simulink model "gm_parallel_8_min_cost_function"  (R2022a)
settings: Solver=FixedStepDiscrete  StartTime=0.0  StopTime=10.0  RelTol=1e-3
undefined symbols (not defined in the file or in its folder): f_c
libraries: hdlmdlgenlib x40
(part 1 of 2)
settings Model: Creator=Andre Merx  LastModifiedBy=Andre Merx
settings SolverCC: AlgebraicLoopSolver=TrustRegion
settings DataIOCC: LimitDataPoints=on  SaveOutput=off  SaveTime=off
settings OptimizationCC: BlockReduction=off  ConditionallyExecuteInputs=off  DefaultParameterBehavior=Inlined  LifeSpan=inf
settings DebuggingCC: AlgebraicLoopMsg=error  InheritedTsInSrcMsg=none  SingleTaskRateTransMsg=error  UnconnectedInputMsg=warning  UnconnectedOutputMsg=warning  UnconnectedLineMsg=warning  AllowSymbolicDim=off  StrictBusMsg=ErrorOnBusTreatedAsVector  SFUnexpectedBacktrackingDiag=warning  SFNoUnconditionalDefaultTransitionDiag=warning  SFExecutionAtInitializationDiag=none  SFMachineParentedDataDiag=warning  ArithmeticOperatorsInVariantConditions=warning
settings HardwareCC: ProdBitPerPointer=32  ProdBitPerSizeT=32  ProdBitPerPtrDiffT=32  ProdLargestAtomicFloat=None  ProdIntDivRoundTo=Undefined  ProdEndianess=Unspecified  ProdWordSize=32  ProdHWDeviceType=ASIC/FPGA->ASIC/FPGA  ProdEqTarget=off
settings SFSimCC: SimUseLocalCustomCode=off  CustomCodeUndefinedFunction=UseInterfaceOnly
settings RTWCC: RTWUseLocalCustomCode=off
settings CodeAppCC: StateflowObjectComments=on
settings GRTTargetCC: TargetLangStandard=C89/C90 (ANSI)
settings ConfigComp: CovScope=ReferencedModels  CovMetricSettings=dw  CovSaveCumulativeToWorkspaceVar=on  CovSaveSingleToWorkspaceVar=on  CovExternalEMLEnable=off  CovSFcnEnable=off

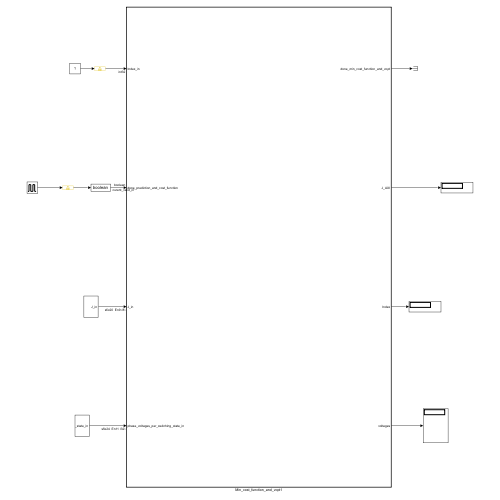
[thumbnail: Simulink's stored preview of the top-level diagram]
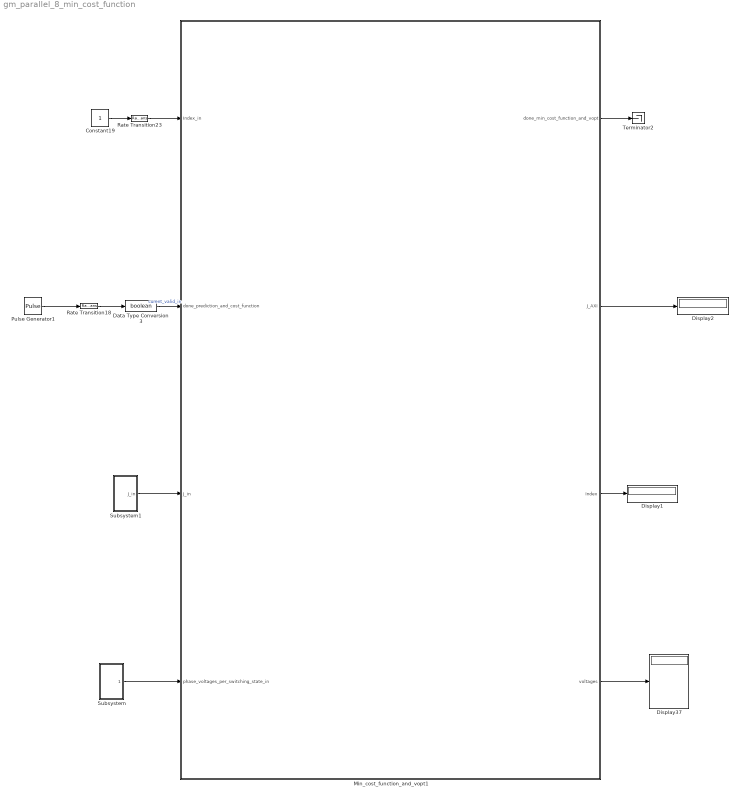
== system gm_parallel_8_min_cost_function ==
  Constant19 : Constant  OutDataTypeStr=int32  SampleTime=-1
  Data Type Conversion3 : DataTypeConversion  OutDataTypeStr=boolean  SaturateOnIntegerOverflow=off  RndMeth=Floor
  Display1 : Display
  Display2 : Display
  Display37 : Display
  Min_cost_function_and_vopt1 : Subsystem  TreatAsAtomicUnit=on
  Pulse Generator1 : DiscretePulseGenerator  PulseType=Time based  Period=1/f_c
  Rate Transition18 : RateTransition  OutPortSampleTime=Rt
  Rate Transition23 : RateTransition  OutPortSampleTime=Rt
  Subsystem : Subsystem
  Subsystem1 : Subsystem
  Terminator2 : Terminator
  wires:
  Min_cost_function_and_vopt1/1(done_min_cost_function_and_vopt) -> Terminator2/1
  Min_cost_function_and_vopt1/2(J_AXI) -> Display2/1
  Min_cost_function_and_vopt1/3(Index) -> Display1/1
  Min_cost_function_and_vopt1/4(voltages) -> Display37/1
  Rate Transition18/1 -> Data Type Conversion3/1
  Pulse Generator1/1 -> Rate Transition18/1
  Data Type Conversion3/1 -> Min_cost_function_and_vopt1/2(done_prediction_and_cost_function)  "curent_valid_in"
  Rate Transition23/1 -> Min_cost_function_and_vopt1/1(Index_in)
  Constant19/1 -> Rate Transition23/1
  Subsystem1/1(J_in) -> Min_cost_function_and_vopt1/3(J_in)
  Subsystem/1(phase_voltages_per_switching_state_in) -> Min_cost_function_and_vopt1/4(phase_voltages_per_switching_state_in)

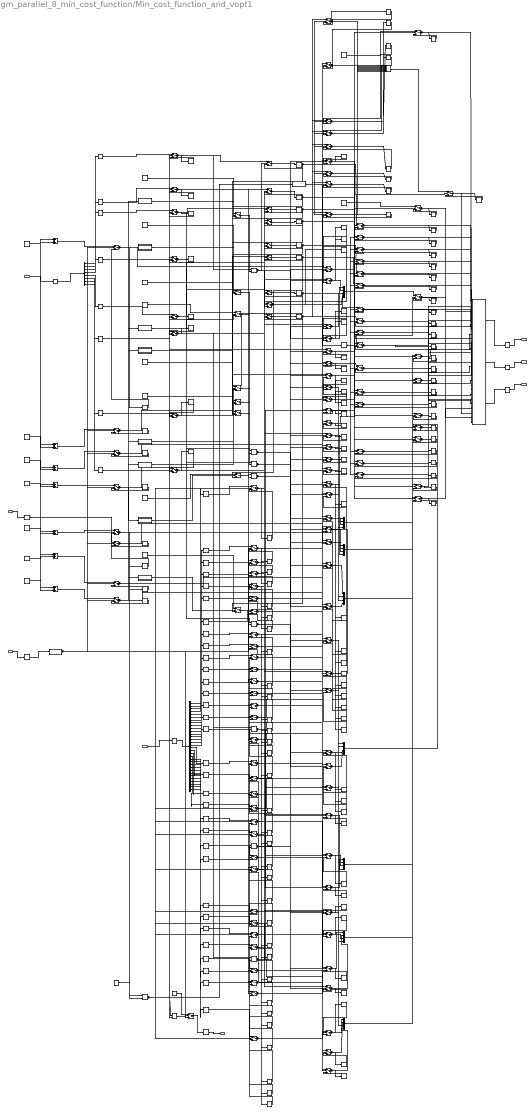
== system gm_parallel_8_min_cost_function/Min_cost_function_and_vopt1 ==
  Index_in : Inport  OutDataTypeStr=int32  PortDimensions=1  SampleTime=1e-08
  done_prediction_and_cost_function : Inport  Port=2  OutDataTypeStr=boolean  PortDimensions=1  SampleTime=1e-08
  J_in : Inport  Port=3  OutDataTypeStr=fixdt(1, 20, 9)  PortDimensions=[8]  SampleTime=1e-08
  phase_voltages_per_switching_state_in : Inport  Port=4  OutDataTypeStr=fixdt(1, 24, 11)  PortDimensions=[32]  SampleTime=1e-08
  Add{,1..6} (7 alike) : Sum  AccumDataTypeStr=fixdt(1, 33, 0)  OutDataTypeStr=fixdt(1, 33, 0)  SampleTime=1e-08
  Compare To Constant : Subsystem  mask(Compare To Constant){relop=<=, const=double(1), OutDataTypeStr=boolean, ZeroCross=on}
      mask prompts: relop "Simulink:masks:Operator_MP"; const "Simulink:masks:ConstantValue_MP"; OutDataTypeStr "Simulink:masks:OutputDataType_MP"; ZeroCross "Simulink:masks:EnableZerocrossingDetection_MP"
      mask help: Simulink:masks:CompareToConstant_MD
      mask init:
      | OutDataTypeStr = 'boolean';
      | ZeroCross = 'on';
      | blkName = 'parallel_8_min_cost_function/Min_cost_function_and_vopt1/Compare\nTo Constant';
      | const = double(1);
      | const_str = '1';
      | const_val = double(1);
      | relop = '<=';
      | setValue = 'boolean';
      | str = '<= 1';
      mask TypeOptions relop: == | ~= | < | <= | >= | >
      mask TypeOptions OutDataTypeStr: Simulink:masks:uint8 | Simulink:masks:boolean
      mask Callback ZeroCross: sl('zeroCrossEnable', gcbh);
      mask Display: disp(str)
  Compare To Constant1 : Subsystem  mask(Compare To Constant){relop=<=, const=double(9), OutDataTypeStr=boolean, ZeroCross=on}
      mask prompts: relop "Simulink:masks:Operator_MP"; const "Simulink:masks:ConstantValue_MP"; OutDataTypeStr "Simulink:masks:OutputDataType_MP"; ZeroCross "Simulink:masks:EnableZerocrossingDetection_MP"
      mask help: Simulink:masks:CompareToConstant_MD
      mask init:
      | OutDataTypeStr = 'boolean';
      | ZeroCross = 'on';
      | blkName = 'parallel_8_min_cost_function/Min_cost_function_and_vopt1/Compare\nTo Constant1';
      | const = double(9);
      | const_str = '9';
      | const_val = double(9);
      | relop = '<=';
      | setValue = 'boolean';
      | str = '<= 9';
      mask TypeOptions relop: == | ~= | < | <= | >= | >
      mask TypeOptions OutDataTypeStr: Simulink:masks:uint8 | Simulink:masks:boolean
      mask Callback ZeroCross: sl('zeroCrossEnable', gcbh);
      mask Display: disp(str)
  Compare To Constant2 : Subsystem  mask(Compare To Constant){relop=<=, const=double(17), OutDataTypeStr=boolean, ZeroCross=on}
      mask prompts: relop "Simulink:masks:Operator_MP"; const "Simulink:masks:ConstantValue_MP"; OutDataTypeStr "Simulink:masks:OutputDataType_MP"; ZeroCross "Simulink:masks:EnableZerocrossingDetection_MP"
      mask help: Simulink:masks:CompareToConstant_MD
      mask init:
      | OutDataTypeStr = 'boolean';
      | ZeroCross = 'on';
      | blkName = 'parallel_8_min_cost_function/Min_cost_function_and_vopt1/Compare\nTo Constant2';
      | const = double(17);
      | const_str = '17';
      | const_val = double(17);
      | relop = '<=';
      | setValue = 'boolean';
      | str = '<= 17';
      mask TypeOptions relop: == | ~= | < | <= | >= | >
      mask TypeOptions OutDataTypeStr: Simulink:masks:uint8 | Simulink:masks:boolean
      mask Callback ZeroCross: sl('zeroCrossEnable', gcbh);
      mask Display: disp(str)
  Compare To Constant3 : Subsystem  mask(Compare To Constant){relop=<=, const=double(25), OutDataTypeStr=boolean, ZeroCross=on}
      mask prompts: relop "Simulink:masks:Operator_MP"; const "Simulink:masks:ConstantValue_MP"; OutDataTypeStr "Simulink:masks:OutputDataType_MP"; ZeroCross "Simulink:masks:EnableZerocrossingDetection_MP"
      mask help: Simulink:masks:CompareToConstant_MD
      mask init:
      | OutDataTypeStr = 'boolean';
      | ZeroCross = 'on';
      | blkName = 'parallel_8_min_cost_function/Min_cost_function_and_vopt1/Compare\nTo Constant3';
      | const = double(25);
      | const_str = '25';
      | const_val = double(25);
      | relop = '<=';
      | setValue = 'boolean';
      | str = '<= 25';
      mask TypeOptions relop: == | ~= | < | <= | >= | >
      mask TypeOptions OutDataTypeStr: Simulink:masks:uint8 | Simulink:masks:boolean
      mask Callback ZeroCross: sl('zeroCrossEnable', gcbh);
      mask Display: disp(str)
  Compare To Constant4 : Subsystem  mask(Compare To Constant){relop=<=, const=double(33), OutDataTypeStr=boolean, ZeroCross=on}
      mask prompts: relop "Simulink:masks:Operator_MP"; const "Simulink:masks:ConstantValue_MP"; OutDataTypeStr "Simulink:masks:OutputDataType_MP"; ZeroCross "Simulink:masks:EnableZerocrossingDetection_MP"
      mask help: Simulink:masks:CompareToConstant_MD
      mask init:
      | OutDataTypeStr = 'boolean';
      | ZeroCross = 'on';
      | blkName = 'parallel_8_min_cost_function/Min_cost_function_and_vopt1/Compare\nTo Constant4';
      | const = double(33);
      | const_str = '33';
      | const_val = double(33);
      | relop = '<=';
      | setValue = 'boolean';
      | str = '<= 33';
      mask TypeOptions relop: == | ~= | < | <= | >= | >
      mask TypeOptions OutDataTypeStr: Simulink:masks:uint8 | Simulink:masks:boolean
      mask Callback ZeroCross: sl('zeroCrossEnable', gcbh);
      mask Display: disp(str)
  Compare To Constant5 : Subsystem  mask(Compare To Constant){relop=<=, const=double(41), OutDataTypeStr=boolean, ZeroCross=on}
      mask prompts: relop "Simulink:masks:Operator_MP"; const "Simulink:masks:ConstantValue_MP"; OutDataTypeStr "Simulink:masks:OutputDataType_MP"; ZeroCross "Simulink:masks:EnableZerocrossingDetection_MP"
      mask help: Simulink:masks:CompareToConstant_MD
      mask init:
      | OutDataTypeStr = 'boolean';
      | ZeroCross = 'on';
      | blkName = 'parallel_8_min_cost_function/Min_cost_function_and_vopt1/Compare\nTo Constant5';
      | const = double(41);
      | const_str = '41';
      | const_val = double(41);
      | relop = '<=';
      | setValue = 'boolean';
      | str = '<= 41';
      mask TypeOptions relop: == | ~= | < | <= | >= | >
      mask TypeOptions OutDataTypeStr: Simulink:masks:uint8 | Simulink:masks:boolean
      mask Callback ZeroCross: sl('zeroCrossEnable', gcbh);
      mask Display: disp(str)
  Compare To Constant6 : Subsystem  mask(Compare To Constant){relop=<=, const=double(49), OutDataTypeStr=boolean, ZeroCross=on}
      mask prompts: relop "Simulink:masks:Operator_MP"; const "Simulink:masks:ConstantValue_MP"; OutDataTypeStr "Simulink:masks:OutputDataType_MP"; ZeroCross "Simulink:masks:EnableZerocrossingDetection_MP"
      mask help: Simulink:masks:CompareToConstant_MD
      mask init:
      | OutDataTypeStr = 'boolean';
      | ZeroCross = 'on';
      | blkName = 'parallel_8_min_cost_function/Min_cost_function_and_vopt1/Compare\nTo Constant6';
      | const = double(49);
      | const_str = '49';
      | const_val = double(49);
      | relop = '<=';
      | setValue = 'boolean';
      | str = '<= 49';
      mask TypeOptions relop: == | ~= | < | <= | >= | >
      mask TypeOptions OutDataTypeStr: Simulink:masks:uint8 | Simulink:masks:boolean
      mask Callback ZeroCross: sl('zeroCrossEnable', gcbh);
      mask Display: disp(str)
  Compare To Constant7 : Subsystem  mask(Compare To Constant){relop=<=, const=double(57), OutDataTypeStr=boolean, ZeroCross=on}
      mask prompts: relop "Simulink:masks:Operator_MP"; const "Simulink:masks:ConstantValue_MP"; OutDataTypeStr "Simulink:masks:OutputDataType_MP"; ZeroCross "Simulink:masks:EnableZerocrossingDetection_MP"
      mask help: Simulink:masks:CompareToConstant_MD
      mask init:
      | OutDataTypeStr = 'boolean';
      | ZeroCross = 'on';
      | blkName = 'parallel_8_min_cost_function/Min_cost_function_and_vopt1/Compare\nTo Constant7';
      | const = double(57);
      | const_str = '57';
      | const_val = double(57);
      | relop = '<=';
      | setValue = 'boolean';
      | str = '<= 57';
      mask TypeOptions relop: == | ~= | < | <= | >= | >
      mask TypeOptions OutDataTypeStr: Simulink:masks:uint8 | Simulink:masks:boolean
      mask Callback ZeroCross: sl('zeroCrossEnable', gcbh);
      mask Display: disp(str)
  Constant{,3..9} (8 alike) : Constant  Value=1000  OutDataTypeStr=fixdt(1, 20, 9)  SampleTime=1e-08
  Constant1 : Constant  Value=8  OutDataTypeStr=int32  SampleTime=1e-08
  Constant10 : Constant  Value=0  OutDataTypeStr=fixdt(1, 20, 9)  SampleTime=1e-08
  Constant11 : Constant  Value="repmat(0,[4  1])"  OutDataTypeStr=fixdt(1, 24, 11)  SampleTime=1e-08
  Constant18 : Constant  Value=8  OutDataTypeStr=int32  SampleTime=1e-08
  Constant19 : Constant  Value=16  OutDataTypeStr=int32  SampleTime=1e-08
  Constant2 : Constant  Value=0  OutDataTypeStr=boolean  SampleTime=1e-08
  Constant20 : Constant  Value=24  OutDataTypeStr=int32  SampleTime=1e-08
  Constant21 : Constant  Value=32  OutDataTypeStr=int32  SampleTime=1e-08
  Constant22 : Constant  Value=40  OutDataTypeStr=int32  SampleTime=1e-08
  Constant23 : Constant  Value=48  OutDataTypeStr=int32  SampleTime=1e-08
  Constant24 : Constant  Value=56  OutDataTypeStr=int32  SampleTime=1e-08
  Delay{,1..9,11..73,81..90,95..96,104..113,118..119,127..136,141..142,150..159,164..165,173..182,371..378} (139 alike) : Delay  DelayLength=double(1)  InitialCondition=0  SampleTime=1e-08
  Delay74 : Delay  DelayLength=double(2)  InitialCondition=0  SampleTime=1e-08
  Delay7_out1_0_wire : hdlmdlgenlib/Buffer
      settings: SourceProductBaseCode=SL
  Delay7_out1_1_wire : hdlmdlgenlib/Buffer
      settings: SourceProductBaseCode=SL
  Delay7_out1_2_wire : hdlmdlgenlib/Buffer
      settings: SourceProductBaseCode=SL
  Delay7_out1_3_wire : hdlmdlgenlib/Buffer
      settings: SourceProductBaseCode=SL
  Delay7_out1_4_wire : hdlmdlgenlib/Buffer
      settings: SourceProductBaseCode=SL
  Delay7_out1_5_wire : hdlmdlgenlib/Buffer
      settings: SourceProductBaseCode=SL
  Delay7_out1_6_wire : hdlmdlgenlib/Buffer
      settings: SourceProductBaseCode=SL
  Delay7_out1_7_wire : hdlmdlgenlib/Buffer
      settings: SourceProductBaseCode=SL
  Delay8_out1_0_wire : hdlmdlgenlib/Buffer
      settings: SourceProductBaseCode=SL
  Delay8_out1_10_wire : hdlmdlgenlib/Buffer
      settings: SourceProductBaseCode=SL
  Delay8_out1_11_wire : hdlmdlgenlib/Buffer
      settings: SourceProductBaseCode=SL
  Delay8_out1_12_wire : hdlmdlgenlib/Buffer
      settings: SourceProductBaseCode=SL
  Delay8_out1_13_wire : hdlmdlgenlib/Buffer
      settings: SourceProductBaseCode=SL
  Delay8_out1_14_wire : hdlmdlgenlib/Buffer
      settings: SourceProductBaseCode=SL
  Delay8_out1_15_wire : hdlmdlgenlib/Buffer
      settings: SourceProductBaseCode=SL
  Delay8_out1_16_wire : hdlmdlgenlib/Buffer
      settings: SourceProductBaseCode=SL
  Delay8_out1_17_wire : hdlmdlgenlib/Buffer
      settings: SourceProductBaseCode=SL
  Delay8_out1_18_wire : hdlmdlgenlib/Buffer
      settings: SourceProductBaseCode=SL
  Delay8_out1_19_wire : hdlmdlgenlib/Buffer
      settings: SourceProductBaseCode=SL
  Delay8_out1_1_wire : hdlmdlgenlib/Buffer
      settings: SourceProductBaseCode=SL
  Delay8_out1_20_wire : hdlmdlgenlib/Buffer
      settings: SourceProductBaseCode=SL
  Delay8_out1_21_wire : hdlmdlgenlib/Buffer
      settings: SourceProductBaseCode=SL
  Delay8_out1_22_wire : hdlmdlgenlib/Buffer
      settings: SourceProductBaseCode=SL
  Delay8_out1_23_wire : hdlmdlgenlib/Buffer
      settings: SourceProductBaseCode=SL
  Delay8_out1_24_wire : hdlmdlgenlib/Buffer
      settings: SourceProductBaseCode=SL
  Delay8_out1_25_wire : hdlmdlgenlib/Buffer
      settings: SourceProductBaseCode=SL
  Delay8_out1_26_wire : hdlmdlgenlib/Buffer
      settings: SourceProductBaseCode=SL
  Delay8_out1_27_wire : hdlmdlgenlib/Buffer
      settings: SourceProductBaseCode=SL
  Delay8_out1_28_wire : hdlmdlgenlib/Buffer
      settings: SourceProductBaseCode=SL
  Delay8_out1_29_wire : hdlmdlgenlib/Buffer
      settings: SourceProductBaseCode=SL
  Delay8_out1_2_wire : hdlmdlgenlib/Buffer
      settings: SourceProductBaseCode=SL
  Delay8_out1_30_wire : hdlmdlgenlib/Buffer
      settings: SourceProductBaseCode=SL
  Delay8_out1_31_wire : hdlmdlgenlib/Buffer
      settings: SourceProductBaseCode=SL
  Delay8_out1_3_wire : hdlmdlgenlib/Buffer
      settings: SourceProductBaseCode=SL
  Delay8_out1_4_wire : hdlmdlgenlib/Buffer
      settings: SourceProductBaseCode=SL
  Delay8_out1_5_wire : hdlmdlgenlib/Buffer
      settings: SourceProductBaseCode=SL
  Delay8_out1_6_wire : hdlmdlgenlib/Buffer
      settings: SourceProductBaseCode=SL
  Delay8_out1_7_wire : hdlmdlgenlib/Buffer
      settings: SourceProductBaseCode=SL
  Delay8_out1_8_wire : hdlmdlgenlib/Buffer
      settings: SourceProductBaseCode=SL
  Delay8_out1_9_wire : hdlmdlgenlib/Buffer
      settings: SourceProductBaseCode=SL
  Detect Rise Positive : Subsystem  mask(Detect Rise Positive){vinit=double(0), InputProcessing=Elements as channels (sample based), OutDataTypeStr=boolean}
      mask prompts: vinit "Simulink:masks:InitialCondition_MP"; InputProcessing "Simulink:masks:InputProcessing_MP"; OutDataTypeStr "Simulink:masks:OutputDataType_MP"
      mask help: Simulink:masks:DetectRisePositive_MD
      mask init:
      | InputProcessing = 'Elements as channels (sample based)';
      | OutDataTypeStr = 'boolean';
      | vinit = double(0);
      mask TypeOptions InputProcessing: Simulink:masks:ColumnsAsChannelsFrameBased | Simulink:masks:ElementsAsChannelsSampleBased
      mask TypeOptions OutDataTypeStr: Simulink:masks:uint8 | Simulink:masks:boolean
      mask Display: fprintf('U > 0\n&  NOT\nU/z > 0')
  Detect Rise Positive1 : Subsystem  mask(Detect Rise Positive){vinit=double(0), InputProcessing=Elements as channels (sample based), OutDataTypeStr=boolean}
      mask prompts: vinit "Simulink:masks:InitialCondition_MP"; InputProcessing "Simulink:masks:InputProcessing_MP"; OutDataTypeStr "Simulink:masks:OutputDataType_MP"
      mask help: Simulink:masks:DetectRisePositive_MD
      mask init:
      | InputProcessing = 'Elements as channels (sample based)';
      | OutDataTypeStr = 'boolean';
      | vinit = double(0);
      mask TypeOptions InputProcessing: Simulink:masks:ColumnsAsChannelsFrameBased | Simulink:masks:ElementsAsChannelsSampleBased
      mask TypeOptions OutDataTypeStr: Simulink:masks:uint8 | Simulink:masks:boolean
      mask Display: fprintf('U > 0\n&  NOT\nU/z > 0')
  Logical Operator : Logic  AllPortsSameDT=off  OutDataTypeStr=boolean  SampleTime=1e-08
  MATLAB Function : Subsystem
  MinMax : MinMax  Inputs=8  ZeroCross=off
  Relational Operator{,2..8} (8 alike) : RelationalOperator  Operator=<  OutDataTypeStr=boolean  SampleTime=1e-08  InputSameDT=off
  Relational Operator1 : RelationalOperator  Operator===  OutDataTypeStr=boolean  SampleTime=1e-08  InputSameDT=off
  Switch{,1,8..9,20..21,27..28,34..35,41..42,48..49,55..56} (16 alike) : Switch  Criteria=u2 > Threshold  Threshold=double(0)  OutDataTypeStr=fixdt(1, 20, 9)  SampleTime=1e-08  SaturateOnIntegerOverflow=off  InputSameDT=off
  Switch{2,10,15,22,29,36,43,50} (8 alike) : Switch  Criteria=u2 > Threshold  Threshold=double(0)  OutDataTypeStr=int32  SampleTime=1e-08  SaturateOnIntegerOverflow=off  InputSameDT=off
  Switch{3..6,11..14,16..19,23..26,30..33,37..40,44..47,51..54} (32 alike) : Switch  Criteria=u2 > Threshold  Threshold=double(0)  OutDataTypeStr=fixdt(1, 24, 11)  SampleTime=1e-08  SaturateOnIntegerOverflow=off  InputSameDT=off
  Switch7 : Switch  Criteria=u2 > Threshold  Threshold=double(0)  OutDataTypeStr=boolean  SampleTime=1e-08  SaturateOnIntegerOverflow=off  InputSameDT=off
  Switch_on{1,53,56,59,62,65,68,71,74} (9 alike) : Switch  Threshold=double(1)  OutDataTypeStr=int32  RndMeth=Simplest  SampleTime=1e-08  SaturateOnIntegerOverflow=off  InputSameDT=off
  Switch_on{4,10,14,20,26,32,38,44,50..51,54,57,60,63,66,69,72,75,98..105} (26 alike) : Switch  Threshold=double(1)  OutDataTypeStr=fixdt(1, 20, 9)  RndMeth=Simplest  SampleTime=1e-08  SaturateOnIntegerOverflow=off  InputSameDT=off
  Switch_on{2..3,5..6,8..9,11..13,15..16,18..19,21..22,24..25,27..28,30..31,33..34,36..37,39..40,42..43,45..46,48..49,52,55,58,61,64,67,70,73} (41 alike) : Switch  Threshold=double(1)  OutDataTypeStr=fixdt(1, 24, 11)  RndMeth=Simplest  SampleTime=1e-08  SaturateOnIntegerOverflow=off  InputSameDT=off
  Switch_on{7,17,23,29,35,41,47} (7 alike) : Switch  Threshold=double(1)  OutDataTypeStr=fixdt(1, 33, 0)  RndMeth=Simplest  SampleTime=1e-08  SaturateOnIntegerOverflow=off  InputSameDT=off
  mux{,1..7} (8 alike) : Mux
  t : Demux  Outputs=8
  t1 : Demux  Outputs=32
  done_min_cost_function_and_vopt : Outport  SampleTime=1e-08
  J_AXI : Outport  Port=2  SampleTime=1e-08
  Index : Outport  Port=3  SampleTime=1e-08
  voltages : Outport  Port=4  SampleTime=1e-08
  wires:
  Index_in/1 -> Delay9/1
  done_prediction_and_cost_function/1 -> Delay6/1
  J_in/1 -> Delay7/1
  phase_voltages_per_switching_state_in/1 -> Delay8/1
  Add/1 -> Switch_on7/1
  Add1/1 -> Switch_on17/1
  Add2/1 -> Switch_on23/1
  Add3/1 -> Switch_on29/1
  Add4/1 -> Switch_on35/1
  Add5/1 -> Switch_on41/1
  Add6/1 -> Switch_on47/1
  Compare To Constant/1(y) -> Switch/2
  Compare To Constant1/1(y) -> Switch8/2
  Compare To Constant2/1(y) -> Switch20/2
  Compare To Constant3/1(y) -> Switch27/2
  Compare To Constant4/1(y) -> Switch34/2
  Compare To Constant5/1(y) -> Switch41/2
  Compare To Constant6/1(y) -> Switch48/2
  Compare To Constant7/1(y) -> Switch55/2
  Constant/1 -> Switch/1
  Constant1/1 -> Relational Operator1/1
  Constant10/1 -> Switch_on50/1
  Constant11/1 -> Switch_on13/1
  Constant18/1 -> Add/2
  Constant19/1 -> Add1/2
  Constant2/1 -> Switch7/1
  Constant20/1 -> Add2/2
  Constant21/1 -> Add3/2
  Constant22/1 -> Add4/2
  Constant23/1 -> Add5/2
  Constant24/1 -> Add6/2
  Constant3/1 -> Switch8/1
  Constant4/1 -> Switch20/1
  Constant5/1 -> Switch27/1
  Constant6/1 -> Switch34/1
  Constant7/1 -> Switch41/1
  Constant8/1 -> Switch48/1
  Constant9/1 -> Switch55/1
  Delay/1 -> Switch_on98/1, Switch_on75/1, Switch1/3, Switch/3
  Delay1/1 -> Switch2/3
  Delay104/1 -> Switch_on26/3
  Delay105/1 -> Switch_on29/3
  Delay106/1 -> Switch_on30/3
  Delay107/1 -> Switch30/3
  Delay108/1 -> Switch_on31/3
  Delay109/1 -> Switch_on27/3
  Delay11/1 -> done_min_cost_function_and_vopt/1
  Delay110/1 -> Switch_on28/3
  Delay111/1 -> Switch31/3
  Delay112/1 -> Switch32/3
  Delay113/1 -> Switch33/3
  Delay118/1 -> Switch_on60/1, Switch_on105/1, Switch42/3, Switch41/3
  Delay119/1 -> Switch36/3
  Delay12/1 -> voltages/1
  Delay127/1 -> Switch_on32/3
  Delay128/1 -> Switch_on35/3
  Delay129/1 -> Switch_on36/3
  Delay13/1 -> Index/1
  Delay130/1 -> Switch37/3
  Delay131/1 -> Switch_on37/3
  Delay132/1 -> Switch_on33/3
  Delay133/1 -> Switch_on34/3
  Delay134/1 -> Switch38/3
  Delay135/1 -> Switch39/3
  Delay136/1 -> Switch40/3
  Delay14/1 -> J_AXI/1
  Delay141/1 -> Switch_on57/1, Switch_on102/1, Switch49/3, Switch48/3
  Delay142/1 -> Switch43/3
  Delay15/1 -> Switch_on13/3
  Delay150/1 -> Switch_on38/3
  Delay151/1 -> Switch_on41/3
  Delay152/1 -> Switch_on42/3
  Delay153/1 -> Switch44/3
  Delay154/1 -> Switch_on43/3
  Delay155/1 -> Switch_on39/3
  Delay156/1 -> Switch_on40/3
  Delay157/1 -> Switch45/3
  Delay158/1 -> Switch46/3
  Delay159/1 -> Switch47/3
  Delay16/1 -> Switch_on50/3
  Delay164/1 -> Switch_on54/1, Switch_on103/1, Switch56/3, Switch55/3
  Delay165/1 -> Switch50/3
  Delay17/1 -> Switch_on4/3
  Delay173/1 -> Switch_on44/3
  Delay174/1 -> Switch_on47/3
  Delay175/1 -> Switch_on48/3
  Delay176/1 -> Switch51/3
  Delay177/1 -> Switch_on49/3
  Delay178/1 -> Switch_on45/3
  Delay179/1 -> Switch_on46/3
  Delay18/1 -> Switch_on1/3
  Delay180/1 -> Switch52/3
  Delay181/1 -> Switch53/3
  Delay182/1 -> Switch54/3
  Delay19/1 -> Switch_on2/3
  Delay2/1 -> Switch3/3
  Delay20/1 -> Switch_on3/3
  Delay21/1 -> Switch_on5/3
  Delay22/1 -> Switch_on6/3
  Delay23/1 -> Switch_on51/3
  Delay24/1 -> Switch_on52/3
  Delay25/1 -> Switch_on99/1, Switch_on72/1, Switch9/3, Switch8/3
  Delay26/1 -> Switch10/3
  Delay27/1 -> Switch_on53/3
  Delay28/1 -> Switch_on54/3
  Delay29/1 -> Switch_on55/3
  Delay3/1 -> Switch4/3
  Delay30/1 -> Switch_on56/3
  Delay31/1 -> Switch_on57/3
  Delay32/1 -> Switch_on58/3
  Delay33/1 -> Switch_on59/3
  Delay34/1 -> Switch_on10/3
  Delay35/1 -> Switch_on7/3
  Delay36/1 -> Switch_on8/3
  Delay37/1 -> Switch11/3
  Delay371/1 -> Switch_on98/3
  Delay372/1 -> Switch_on99/3
  Delay373/1 -> Switch_on100/3
  Delay374/1 -> Switch_on101/3
  Delay375/1 -> Switch_on104/3
  Delay376/1 -> Switch_on105/3
  Delay377/1 -> Switch_on102/3
  Delay378/1 -> Switch_on103/3
  Delay38/1 -> Switch_on9/3
  Delay39/1 -> Switch_on11/3
  Delay4/1 -> Switch5/3
  Delay40/1 -> Switch_on12/3
  Delay41/1 -> Switch12/3
  Delay42/1 -> Switch13/3
  Delay43/1 -> Switch14/3
  Delay44/1 -> Switch_on60/3
  Delay45/1 -> Switch_on61/3
  Delay46/1 -> Switch_on62/3
  Delay47/1 -> Switch_on63/3
  Delay48/1 -> Switch_on64/3
  Delay49/1 -> Switch_on69/1, Switch_on100/1, Switch21/3, Switch20/3
  Delay5/1 -> Switch6/3
  Delay50/1 -> Switch15/3
  Delay51/1 -> Switch_on65/3
  Delay52/1 -> Switch_on66/3
  Delay53/1 -> Switch_on67/3
  Delay54/1 -> Switch_on68/3
  Delay55/1 -> Switch_on69/3
  Delay56/1 -> Switch_on70/3
  Delay57/1 -> Switch_on71/3
  Delay58/1 -> Switch_on14/3
  Delay59/1 -> Switch_on17/3
  Delay6/1 -> Detect Rise Positive/1(U)
  Delay60/1 -> Switch_on18/3
  Delay61/1 -> Switch16/3
  Delay62/1 -> Switch_on19/3
  Delay63/1 -> Switch_on15/3
  Delay64/1 -> Switch_on16/3
  Delay65/1 -> Switch17/3
  Delay66/1 -> Switch18/3
  Delay67/1 -> Switch19/3
  Delay68/1 -> Switch_on72/3
  Delay69/1 -> Switch_on73/3
  Delay7/1 -> t/1
  Delay70/1 -> Switch_on74/3
  Delay71/1 -> Switch_on75/3
  Delay72/1 -> Switch_on66/1, Switch_on101/1, Switch28/3, Switch27/3
  Delay73/1 -> Switch22/3
  Delay74/1 -> Switch_on75/2, Switch_on74/2, Switch_on73/2, Switch_on72/2, Switch_on71/2, Switch_on70/2, Switch_on69/2, Switch_on68/2, Switch_on67/2, Switch_on66/2, Switch_on65/2, Switch_on64/2, Switch_on63/2, Switch_on62/2, Switch_on61/2, Switch_on60/2, Switch_on59/2, Switch_on58/2, Switch_on57/2, Switch_on56/2, Switch_on55/2, Switch_on54/2, Switch_on53/2, Switch_on52/2, Switch_on51/2, Switch_on50/2, Switch_on13/2
  Delay8/1 -> t1/1
  Delay81/1 -> Switch_on20/3
  Delay82/1 -> Switch_on23/3
  Delay83/1 -> Switch_on24/3
  Delay84/1 -> Switch23/3
  Delay85/1 -> Switch_on25/3
  Delay86/1 -> Switch_on21/3
  Delay87/1 -> Switch_on22/3
  Delay88/1 -> Switch24/3
  Delay89/1 -> Switch25/3
  Delay9/1 -> Switch_on1/1, Add6/1, Add5/1, Add4/1, Add3/1, Add2/1, Add1/1, Add/1
  Delay90/1 -> Switch26/3
  Delay95/1 -> Switch_on63/1, Switch_on104/1, Switch35/3, Switch34/3
  Delay96/1 -> Switch29/3
  Delay7_out1_0_wire/1 -> Switch_on4/1
  Delay7_out1_1_wire/1 -> Switch_on10/1
  Delay7_out1_2_wire/1 -> Switch_on14/1
  Delay7_out1_3_wire/1 -> Switch_on20/1
  Delay7_out1_4_wire/1 -> Switch_on26/1
  Delay7_out1_5_wire/1 -> Switch_on32/1
  Delay7_out1_6_wire/1 -> Switch_on38/1
  Delay7_out1_7_wire/1 -> Switch_on44/1
  Delay8_out1_0_wire/1 -> Switch_on2/1
  Delay8_out1_1_wire/1 -> Switch_on3/1
  Delay8_out1_2_wire/1 -> Switch_on5/1
  Delay8_out1_3_wire/1 -> Switch_on6/1
  Delay8_out1_4_wire/1 -> Switch_on8/1
  Delay8_out1_5_wire/1 -> Switch_on9/1
  Delay8_out1_6_wire/1 -> Switch_on11/1
  Delay8_out1_7_wire/1 -> Switch_on12/1
  Delay8_out1_8_wire/1 -> Switch_on18/1
  Delay8_out1_9_wire/1 -> Switch_on19/1
  Delay8_out1_10_wire/1 -> Switch_on15/1
  Delay8_out1_11_wire/1 -> Switch_on16/1
  Delay8_out1_12_wire/1 -> Switch_on24/1
  Delay8_out1_13_wire/1 -> Switch_on25/1
  Delay8_out1_14_wire/1 -> Switch_on21/1
  Delay8_out1_15_wire/1 -> Switch_on22/1
  Delay8_out1_16_wire/1 -> Switch_on30/1
  Delay8_out1_17_wire/1 -> Switch_on31/1
  Delay8_out1_18_wire/1 -> Switch_on27/1
  Delay8_out1_19_wire/1 -> Switch_on28/1
  Delay8_out1_20_wire/1 -> Switch_on36/1
  Delay8_out1_21_wire/1 -> Switch_on37/1
  Delay8_out1_22_wire/1 -> Switch_on33/1
  Delay8_out1_23_wire/1 -> Switch_on34/1
  Delay8_out1_24_wire/1 -> Switch_on42/1
  Delay8_out1_25_wire/1 -> Switch_on43/1
  Delay8_out1_26_wire/1 -> Switch_on39/1
  Delay8_out1_27_wire/1 -> Switch_on40/1
  Delay8_out1_28_wire/1 -> Switch_on48/1
  Delay8_out1_29_wire/1 -> Switch_on49/1
  Delay8_out1_30_wire/1 -> Switch_on45/1
  Delay8_out1_31_wire/1 -> Switch_on46/1
  Detect Rise Positive/1(Y) -> Switch_on9/2, Switch_on8/2, Switch_on7/2, Switch_on6/2, Switch_on5/2, Switch_on49/2, Switch_on48/2, Switch_on47/2, Switch_on46/2, Switch_on45/2, Switch_on44/2, Switch_on43/2, Switch_on42/2, Switch_on41/2, Switch_on40/2, Switch_on4/2, Switch_on39/2, Switch_on38/2, Switch_on37/2, Switch_on36/2, Switch_on35/2, Switch_on34/2, Switch_on33/2, Switch_on32/2, Switch_on31/2, Switch_on30/2, Switch_on3/2, Switch_on29/2, Switch_on28/2, Switch_on27/2, Switch_on26/2, Switch_on25/2, Switch_on24/2, Switch_on23/2, Switch_on22/2, Switch_on21/2, Switch_on20/2, Switch_on2/2, Switch_on19/2, Switch_on18/2, Switch_on17/2, Switch_on16/2, Switch_on15/2, Switch_on14/2, Switch_on12/2, Switch_on11/2, Switch_on10/2, Switch_on1/2, Switch7/3, Logical Operator/2
  Detect Rise Positive1/1(Y) -> Switch_on99/2, Switch_on98/2, Switch_on105/2, Switch_on104/2, Switch_on103/2, Switch_on102/2, Switch_on101/2, Switch_on100/2, Delay74/1
  Logical Operator/1 -> Switch7/2
  MATLAB Function/1(J) -> Delay14/1
  MATLAB Function/2(Index) -> Delay13/1
  MATLAB Function/3(voltages) -> Delay12/1
  MinMax/1 -> Switch_on51/1
  mux/1 -> Switch_on73/1
  mux1/1 -> Switch_on70/1
  mux2/1 -> Switch_on67/1
  mux3/1 -> Switch_on64/1
  mux4/1 -> Switch_on61/1
  mux5/1 -> Switch_on58/1
  mux6/1 -> Switch_on55/1
  mux7/1 -> Switch_on52/1
  Relational Operator/1 -> Switch6/2, Switch5/2, Switch4/2, Switch3/2, Switch2/2, Switch1/2
  Relational Operator1/1 -> Logical Operator/1, Detect Rise Positive1/1(U)
  Relational Operator2/1 -> Switch9/2, Switch14/2, Switch13/2, Switch12/2, Switch11/2, Switch10/2
  Relational Operator3/1 -> Switch21/2, Switch19/2, Switch18/2, Switch17/2, Switch16/2, Switch15/2
  Relational Operator4/1 -> Switch28/2, Switch26/2, Switch25/2, Switch24/2, Switch23/2, Switch22/2
  Relational Operator5/1 -> Switch35/2, Switch33/2, Switch32/2, Switch31/2, Switch30/2, Switch29/2
  Relational Operator6/1 -> Switch42/2, Switch40/2, Switch39/2, Switch38/2, Switch37/2, Switch36/2
  Relational Operator7/1 -> Switch49/2, Switch47/2, Switch46/2, Switch45/2, Switch44/2, Switch43/2
  Relational Operator8/1 -> Switch56/2, Switch54/2, Switch53/2, Switch52/2, Switch51/2, Switch50/2
  Switch/1 -> Relational Operator/2
  Switch1/1 -> Delay/1
  Switch10/1 -> Switch_on71/1, Delay26/1
  Switch11/1 -> mux1/1, Delay37/1
  Switch12/1 -> mux1/2, Delay41/1
  Switch13/1 -> mux1/3, Delay42/1
  Switch14/1 -> mux1/4, Delay43/1
  Switch15/1 -> Switch_on68/1, Delay50/1
  Switch16/1 -> mux2/1, Delay61/1
  Switch17/1 -> mux2/2, Delay65/1
  Switch18/1 -> mux2/3, Delay66/1
  Switch19/1 -> mux2/4, Delay67/1
  Switch2/1 -> Switch_on74/1, Delay1/1
  Switch20/1 -> Relational Operator3/2
  Switch21/1 -> Delay49/1
  Switch22/1 -> Switch_on65/1, Delay73/1
  Switch23/1 -> mux3/1, Delay84/1
  Switch24/1 -> mux3/2, Delay88/1
  Switch25/1 -> mux3/3, Delay89/1
  Switch26/1 -> mux3/4, Delay90/1
  Switch27/1 -> Relational Operator4/2
  Switch28/1 -> Delay72/1
  Switch29/1 -> Switch_on62/1, Delay96/1
  Switch3/1 -> mux/1, Delay2/1
  Switch30/1 -> mux4/1, Delay107/1
  Switch31/1 -> mux4/2, Delay111/1
  Switch32/1 -> mux4/3, Delay112/1
  Switch33/1 -> mux4/4, Delay113/1
  Switch34/1 -> Relational Operator5/2
  Switch35/1 -> Delay95/1
  Switch36/1 -> Switch_on59/1, Delay119/1
  Switch37/1 -> mux5/1, Delay130/1
  Switch38/1 -> mux5/2, Delay134/1
  Switch39/1 -> mux5/3, Delay135/1
  Switch4/1 -> mux/2, Delay3/1
  Switch40/1 -> mux5/4, Delay136/1
  Switch41/1 -> Relational Operator6/2
  Switch42/1 -> Delay118/1
  Switch43/1 -> Switch_on56/1, Delay142/1
  Switch44/1 -> mux6/1, Delay153/1
  Switch45/1 -> mux6/2, Delay157/1
  Switch46/1 -> mux6/3, Delay158/1
  Switch47/1 -> mux6/4, Delay159/1
  Switch48/1 -> Relational Operator7/2
  Switch49/1 -> Delay141/1
  Switch5/1 -> mux/3, Delay4/1
  Switch50/1 -> Switch_on53/1, Delay165/1
  Switch51/1 -> mux7/1, Delay176/1
  Switch52/1 -> mux7/2, Delay180/1
  Switch53/1 -> mux7/3, Delay181/1
  Switch54/1 -> mux7/4, Delay182/1
  Switch55/1 -> Relational Operator8/2
  Switch56/1 -> Delay164/1
  Switch6/1 -> mux/4, Delay5/1
  Switch7/1 -> Delay11/1
  Switch8/1 -> Relational Operator2/2
  Switch9/1 -> Delay25/1
  Switch_on1/1 -> Switch2/1, Relational Operator1/2, Delay18/1, Compare To Constant/1(u)
  Switch_on10/1 -> Switch9/1, Relational Operator2/1, Delay34/1
  Switch_on100/1 -> Delay373/1, MinMax/3
  Switch_on101/1 -> Delay374/1, MinMax/4
  Switch_on102/1 -> Delay377/1, MinMax/7
  Switch_on103/1 -> Delay378/1, MinMax/8
  Switch_on104/1 -> Delay375/1, MinMax/5
  Switch_on105/1 -> Delay376/1, MinMax/6
  Switch_on11/1 -> Switch13/1, Delay39/1
  Switch_on12/1 -> Switch14/1, Delay40/1
  Switch_on13/1 -> Delay15/1, MATLAB Function/27(voltages_default)
  Switch_on14/1 -> Switch21/1, Relational Operator3/1, Delay58/1
  Switch_on15/1 -> Switch18/1, Delay63/1
  Switch_on16/1 -> Switch19/1, Delay64/1
  Switch_on17/1 -> Switch15/1, Delay59/1, Compare To Constant2/1(u)
  Switch_on18/1 -> Switch16/1, Delay60/1
  Switch_on19/1 -> Switch17/1, Delay62/1
  Switch_on2/1 -> Switch3/1, Delay19/1
  Switch_on20/1 -> Switch28/1, Relational Operator4/1, Delay81/1
  Switch_on21/1 -> Switch25/1, Delay86/1
  Switch_on22/1 -> Switch26/1, Delay87/1
  Switch_on23/1 -> Switch22/1, Delay82/1, Compare To Constant3/1(u)
  Switch_on24/1 -> Switch23/1, Delay83/1
  Switch_on25/1 -> Switch24/1, Delay85/1
  Switch_on26/1 -> Switch35/1, Relational Operator5/1, Delay104/1
  Switch_on27/1 -> Switch32/1, Delay109/1
  Switch_on28/1 -> Switch33/1, Delay110/1
  Switch_on29/1 -> Switch29/1, Delay105/1, Compare To Constant4/1(u)
  Switch_on3/1 -> Switch4/1, Delay20/1
  Switch_on30/1 -> Switch30/1, Delay106/1
  Switch_on31/1 -> Switch31/1, Delay108/1
  Switch_on32/1 -> Switch42/1, Relational Operator6/1, Delay127/1
  Switch_on33/1 -> Switch39/1, Delay132/1
  Switch_on34/1 -> Switch40/1, Delay133/1
  Switch_on35/1 -> Switch36/1, Delay128/1, Compare To Constant5/1(u)
  Switch_on36/1 -> Switch37/1, Delay129/1
  Switch_on37/1 -> Switch38/1, Delay131/1
  Switch_on38/1 -> Switch49/1, Relational Operator7/1, Delay150/1
  Switch_on39/1 -> Switch46/1, Delay155/1
  Switch_on4/1 -> Switch1/1, Relational Operator/1, Delay17/1
  Switch_on40/1 -> Switch47/1, Delay156/1
  Switch_on41/1 -> Switch43/1, Delay151/1, Compare To Constant6/1(u)
  Switch_on42/1 -> Switch44/1, Delay152/1
  Switch_on43/1 -> Switch45/1, Delay154/1
  Switch_on44/1 -> Switch56/1, Relational Operator8/1, Delay173/1
  Switch_on45/1 -> Switch53/1, Delay178/1
  Switch_on46/1 -> Switch54/1, Delay179/1
  Switch_on47/1 -> Switch50/1, Delay174/1, Compare To Constant7/1(u)
  Switch_on48/1 -> Switch51/1, Delay175/1
  Switch_on49/1 -> Switch52/1, Delay177/1
  Switch_on5/1 -> Switch5/1, Delay21/1
  Switch_on50/1 -> Delay16/1, MATLAB Function/26(J_default)
  Switch_on51/1 -> Delay23/1, MATLAB Function/25(min)
  Switch_on52/1 -> Delay24/1, MATLAB Function/24(voltages_8)
  Switch_on53/1 -> Delay27/1, MATLAB Function/23(Index_8)
  Switch_on54/1 -> Delay28/1, MATLAB Function/22(J_8)
  Switch_on55/1 -> Delay29/1, MATLAB Function/21(voltages_7)
  Switch_on56/1 -> Delay30/1, MATLAB Function/20(Index_7)
  Switch_on57/1 -> Delay31/1, MATLAB Function/19(J_7)
  Switch_on58/1 -> Delay32/1, MATLAB Function/18(voltages_6)
  Switch_on59/1 -> Delay33/1, MATLAB Function/17(Index_6)
  Switch_on6/1 -> Switch6/1, Delay22/1
  Switch_on60/1 -> Delay44/1, MATLAB Function/16(J_6)
  Switch_on61/1 -> Delay45/1, MATLAB Function/15(voltages_5)
  Switch_on62/1 -> Delay46/1, MATLAB Function/14(Index_5)
  Switch_on63/1 -> Delay47/1, MATLAB Function/13(J_5)
  Switch_on64/1 -> Delay48/1, MATLAB Function/12(voltages_4)
  Switch_on65/1 -> Delay51/1, MATLAB Function/11(Index_4)
  Switch_on66/1 -> Delay52/1, MATLAB Function/10(J_4)
  Switch_on67/1 -> Delay53/1, MATLAB Function/9(voltages_3)
  Switch_on68/1 -> Delay54/1, MATLAB Function/8(Index_3)
  Switch_on69/1 -> Delay55/1, MATLAB Function/7(J_3)
  Switch_on7/1 -> Switch10/1, Delay35/1, Compare To Constant1/1(u)
  Switch_on70/1 -> Delay56/1, MATLAB Function/6(voltages_2)
  Switch_on71/1 -> Delay57/1, MATLAB Function/5(Index_2)
  Switch_on72/1 -> Delay68/1, MATLAB Function/4(J_2)
  Switch_on73/1 -> Delay69/1, MATLAB Function/3(voltages_1)
  Switch_on74/1 -> Delay70/1, MATLAB Function/2(Index_1)
  Switch_on75/1 -> Delay71/1, MATLAB Function/1(J_1)
  Switch_on8/1 -> Switch11/1, Delay36/1
  Switch_on9/1 -> Switch12/1, Delay38/1
  Switch_on98/1 -> Delay371/1, MinMax/1
  Switch_on99/1 -> Delay372/1, MinMax/2
  t/1 -> Delay7_out1_0_wire/1
  t/2 -> Delay7_out1_1_wire/1
  t/3 -> Delay7_out1_2_wire/1
  t/4 -> Delay7_out1_3_wire/1
  t/5 -> Delay7_out1_4_wire/1
  t/6 -> Delay7_out1_5_wire/1
  t/7 -> Delay7_out1_6_wire/1
  t/8 -> Delay7_out1_7_wire/1
  t1/1 -> Delay8_out1_0_wire/1
  t1/2 -> Delay8_out1_1_wire/1
  t1/3 -> Delay8_out1_2_wire/1
  t1/4 -> Delay8_out1_3_wire/1
  t1/5 -> Delay8_out1_4_wire/1
  t1/6 -> Delay8_out1_5_wire/1
  t1/7 -> Delay8_out1_6_wire/1
  t1/8 -> Delay8_out1_7_wire/1
  t1/9 -> Delay8_out1_8_wire/1
  t1/10 -> Delay8_out1_9_wire/1
  t1/11 -> Delay8_out1_10_wire/1
  t1/12 -> Delay8_out1_11_wire/1
  t1/13 -> Delay8_out1_12_wire/1
  t1/14 -> Delay8_out1_13_wire/1
  t1/15 -> Delay8_out1_14_wire/1
  t1/16 -> Delay8_out1_15_wire/1
  t1/17 -> Delay8_out1_16_wire/1
  t1/18 -> Delay8_out1_17_wire/1
  t1/19 -> Delay8_out1_18_wire/1
  t1/20 -> Delay8_out1_19_wire/1
  t1/21 -> Delay8_out1_20_wire/1
  t1/22 -> Delay8_out1_21_wire/1
  t1/23 -> Delay8_out1_22_wire/1
  t1/24 -> Delay8_out1_23_wire/1
  t1/25 -> Delay8_out1_24_wire/1
  t1/26 -> Delay8_out1_25_wire/1
  t1/27 -> Delay8_out1_26_wire/1
  t1/28 -> Delay8_out1_27_wire/1
  t1/29 -> Delay8_out1_28_wire/1
  t1/30 -> Delay8_out1_29_wire/1
  t1/31 -> Delay8_out1_30_wire/1
  t1/32 -> Delay8_out1_31_wire/1

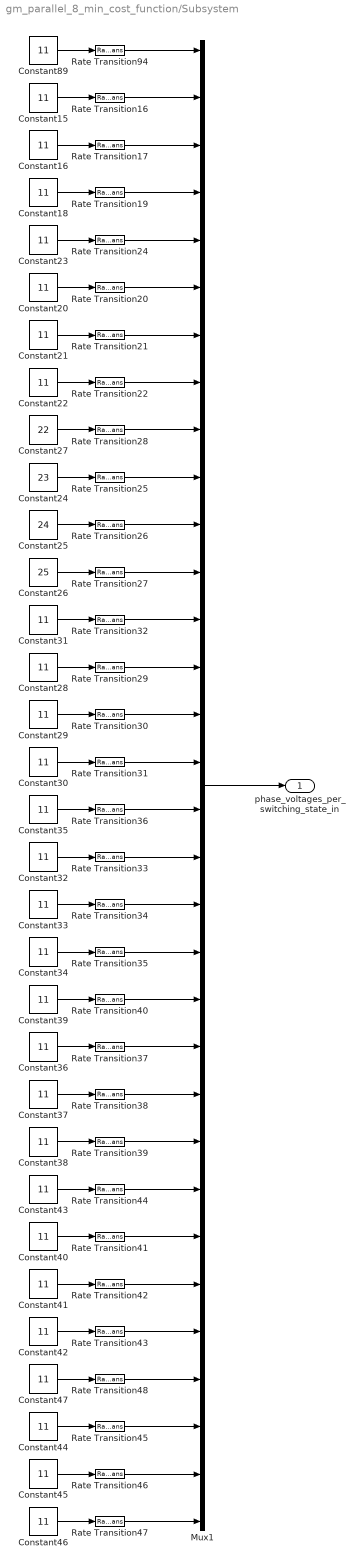
== system gm_parallel_8_min_cost_function/Subsystem ==
  Constant{15..16,18,20..23,28..47,89} (28 alike) : Constant  Value=11  OutDataTypeStr=fixdt(1,24,11)  SampleTime=-1  LockScale=on
  Constant24 : Constant  Value=23  OutDataTypeStr=fixdt(1,24,11)  SampleTime=-1  LockScale=on
  Constant25 : Constant  Value=24  OutDataTypeStr=fixdt(1,24,11)  SampleTime=-1  LockScale=on
  Constant26 : Constant  Value=25  OutDataTypeStr=fixdt(1,24,11)  SampleTime=-1  LockScale=on
  Constant27 : Constant  Value=22  OutDataTypeStr=fixdt(1,24,11)  SampleTime=-1  LockScale=on
  Mux1 : Mux  Inputs=32
  Rate Transition{16..17,19..22,24..48,94} (32 alike) : RateTransition  OutPortSampleTime=Rt
  phase_voltages_per_switching_state_in : Outport  VectorParamsAs1DForOutWhenUnconnected=off
  wires:
  Constant39/1 -> Rate Transition40/1
  Rate Transition41/1 -> Mux1/26
  Rate Transition31/1 -> Mux1/16
  Rate Transition37/1 -> Mux1/22
  Rate Transition35/1 -> Mux1/20
  Rate Transition47/1 -> Mux1/32
  Rate Transition26/1 -> Mux1/11
  Rate Transition46/1 -> Mux1/31
  Rate Transition40/1 -> Mux1/21
  Rate Transition27/1 -> Mux1/12
  Rate Transition20/1 -> Mux1/6
  Rate Transition33/1 -> Mux1/18
  Rate Transition22/1 -> Mux1/8
  Rate Transition21/1 -> Mux1/7
  Rate Transition30/1 -> Mux1/15
  Rate Transition19/1 -> Mux1/4
  Constant38/1 -> Rate Transition39/1
  Rate Transition29/1 -> Mux1/14
  Rate Transition42/1 -> Mux1/27
  Constant40/1 -> Rate Transition41/1
  Constant25/1 -> Rate Transition26/1
  Constant26/1 -> Rate Transition27/1
  Constant16/1 -> Rate Transition17/1
  Constant45/1 -> Rate Transition46/1
  Constant23/1 -> Rate Transition24/1
  Constant44/1 -> Rate Transition45/1
  Rate Transition43/1 -> Mux1/28
  Constant89/1 -> Rate Transition94/1
  Constant31/1 -> Rate Transition32/1
  Constant15/1 -> Rate Transition16/1
  Rate Transition38/1 -> Mux1/23
  Constant30/1 -> Rate Transition31/1
  Rate Transition44/1 -> Mux1/25
  Constant28/1 -> Rate Transition29/1
  Rate Transition45/1 -> Mux1/30
  Constant21/1 -> Rate Transition21/1
  Rate Transition25/1 -> Mux1/10
  Rate Transition24/1 -> Mux1/5
  Constant46/1 -> Rate Transition47/1
  Constant29/1 -> Rate Transition30/1
  Rate Transition32/1 -> Mux1/13
  Constant22/1 -> Rate Transition22/1
  Constant33/1 -> Rate Transition34/1
  Constant47/1 -> Rate Transition48/1
  Constant27/1 -> Rate Transition28/1
  Constant41/1 -> Rate Transition42/1
  Rate Transition39/1 -> Mux1/24
  Rate Transition17/1 -> Mux1/3
  Constant34/1 -> Rate Transition35/1
  Rate Transition16/1 -> Mux1/2
  Rate Transition28/1 -> Mux1/9
  Constant20/1 -> Rate Transition20/1
  Constant43/1 -> Rate Transition44/1
  Rate Transition48/1 -> Mux1/29
  Constant37/1 -> Rate Transition38/1
  Rate Transition34/1 -> Mux1/19
  Constant36/1 -> Rate Transition37/1
  Rate Transition94/1 -> Mux1/1
  Constant18/1 -> Rate Transition19/1
  Constant32/1 -> Rate Transition33/1
  Constant24/1 -> Rate Transition25/1
  Mux1/1 -> phase_voltages_per_switching_state_in/1
  Constant42/1 -> Rate Transition43/1
  Constant35/1 -> Rate Transition36/1
  Rate Transition36/1 -> Mux1/17

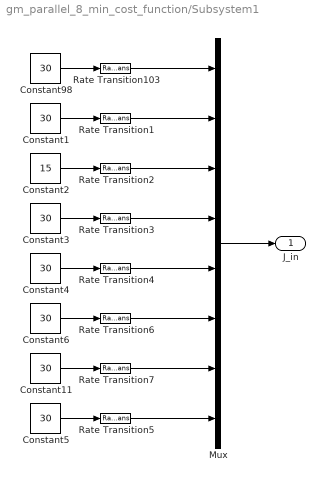
== system gm_parallel_8_min_cost_function/Subsystem1 ==
  Constant{1,3..6,11,98} (7 alike) : Constant  Value=30  OutDataTypeStr=fixdt(1,20,9)  SampleTime=-1
  Constant2 : Constant  Value=15  OutDataTypeStr=fixdt(1,20,9)  SampleTime=-1
  Mux : Mux  Inputs=8
  Rate Transition{1..7,103} (8 alike) : RateTransition  OutPortSampleTime=Rt
  J_in : Outport
  wires:
  Mux/1 -> J_in/1
  Constant6/1 -> Rate Transition6/1
  Rate Transition6/1 -> Mux/6
  Constant2/1 -> Rate Transition2/1
  Constant98/1 -> Rate Transition103/1
  Rate Transition3/1 -> Mux/4
  Constant4/1 -> Rate Transition4/1
  Rate Transition7/1 -> Mux/7
  Constant5/1 -> Rate Transition5/1
  Rate Transition1/1 -> Mux/2
  Constant3/1 -> Rate Transition3/1
  Rate Transition2/1 -> Mux/3
  Rate Transition4/1 -> Mux/5
  Constant11/1 -> Rate Transition7/1
  Rate Transition5/1 -> Mux/8
  Rate Transition103/1 -> Mux/1
  Constant1/1 -> Rate Transition1/1

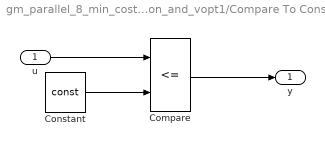
== system gm_parallel_8_min_cost_function/Min_cost_function_and_vopt1/Compare To Constant ==
  u : Inport  OutDataTypeStr=int32  SampleTime=1e-08
  Compare : RelationalOperator  Operator=<=  OutDataTypeStr=boolean
  Constant : Constant  DisableCoverage=on  Value=const  OutDataTypeStr=Inherit: Inherit via back propagation  SampleTime=-1
  y : Outport  SampleTime=1e-08
  wires:
  u/1 -> Compare/1
  Compare/1 -> y/1
  Constant/1 -> Compare/2

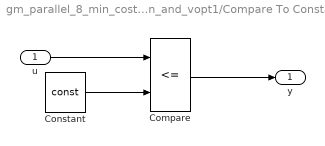
== system gm_parallel_8_min_cost_function/Min_cost_function_and_vopt1/Compare To Constant1 ==
  u : Inport  OutDataTypeStr=fixdt(1, 33, 0)  SampleTime=1e-08
  Compare : RelationalOperator  Operator=<=  OutDataTypeStr=boolean
  Constant : Constant  DisableCoverage=on  Value=const  OutDataTypeStr=Inherit: Inherit via back propagation  SampleTime=-1
  y : Outport  SampleTime=1e-08
  wires:
  u/1 -> Compare/1
  Compare/1 -> y/1
  Constant/1 -> Compare/2

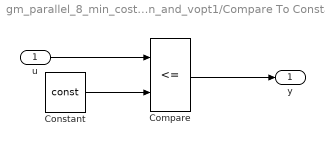
== system gm_parallel_8_min_cost_function/Min_cost_function_and_vopt1/Compare To Constant2 ==
  u : Inport  OutDataTypeStr=fixdt(1, 33, 0)  SampleTime=1e-08
  Compare : RelationalOperator  Operator=<=  OutDataTypeStr=boolean
  Constant : Constant  DisableCoverage=on  Value=const  OutDataTypeStr=Inherit: Inherit via back propagation  SampleTime=-1
  y : Outport  SampleTime=1e-08
  wires:
  u/1 -> Compare/1
  Compare/1 -> y/1
  Constant/1 -> Compare/2

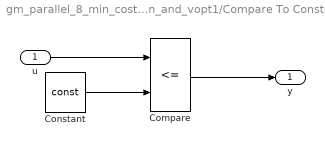
== system gm_parallel_8_min_cost_function/Min_cost_function_and_vopt1/Compare To Constant3 ==
  u : Inport  OutDataTypeStr=fixdt(1, 33, 0)  SampleTime=1e-08
  Compare : RelationalOperator  Operator=<=  OutDataTypeStr=boolean
  Constant : Constant  DisableCoverage=on  Value=const  OutDataTypeStr=Inherit: Inherit via back propagation  SampleTime=-1
  y : Outport  SampleTime=1e-08
  wires:
  u/1 -> Compare/1
  Compare/1 -> y/1
  Constant/1 -> Compare/2

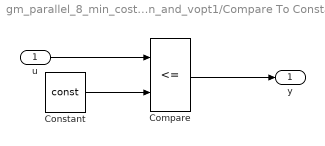
== system gm_parallel_8_min_cost_function/Min_cost_function_and_vopt1/Compare To Constant4 ==
  u : Inport  OutDataTypeStr=fixdt(1, 33, 0)  SampleTime=1e-08
  Compare : RelationalOperator  Operator=<=  OutDataTypeStr=boolean
  Constant : Constant  DisableCoverage=on  Value=const  OutDataTypeStr=Inherit: Inherit via back propagation  SampleTime=-1
  y : Outport  SampleTime=1e-08
  wires:
  u/1 -> Compare/1
  Compare/1 -> y/1
  Constant/1 -> Compare/2

== system gm_parallel_8_min_cost_function/Min_cost_function_and_vopt1/Compare To Constant5 ==
  u : Inport  OutDataTypeStr=fixdt(1, 33, 0)  SampleTime=1e-08
  Compare : RelationalOperator  Operator=<=  OutDataTypeStr=boolean
  Constant : Constant  DisableCoverage=on  Value=const  OutDataTypeStr=Inherit: Inherit via back propagation  SampleTime=-1
  y : Outport  SampleTime=1e-08
  wires:
  u/1 -> Compare/1
  Compare/1 -> y/1
  Constant/1 -> Compare/2

== system gm_parallel_8_min_cost_function/Min_cost_function_and_vopt1/Compare To Constant6 ==
  u : Inport  OutDataTypeStr=fixdt(1, 33, 0)  SampleTime=1e-08
  Compare : RelationalOperator  Operator=<=  OutDataTypeStr=boolean
  Constant : Constant  DisableCoverage=on  Value=const  OutDataTypeStr=Inherit: Inherit via back propagation  SampleTime=-1
  y : Outport  SampleTime=1e-08
  wires:
  u/1 -> Compare/1
  Compare/1 -> y/1
  Constant/1 -> Compare/2

== system gm_parallel_8_min_cost_function/Min_cost_function_and_vopt1/Compare To Constant7 ==
  u : Inport  OutDataTypeStr=fixdt(1, 33, 0)  SampleTime=1e-08
  Compare : RelationalOperator  Operator=<=  OutDataTypeStr=boolean
  Constant : Constant  DisableCoverage=on  Value=const  OutDataTypeStr=Inherit: Inherit via back propagation  SampleTime=-1
  y : Outport  SampleTime=1e-08
  wires:
  u/1 -> Compare/1
  Compare/1 -> y/1
  Constant/1 -> Compare/2

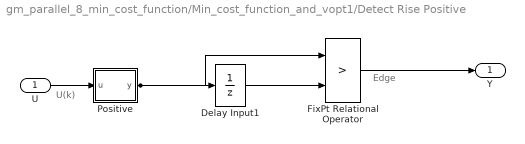
== system gm_parallel_8_min_cost_function/Min_cost_function_and_vopt1/Detect Rise Positive ==
  note: Edge
  note: U(k)
  U : Inport  OutDataTypeStr=boolean  SampleTime=1e-08
  Delay Input1 : UnitDelay  Description=Store in Global RAM  DisableCoverage=on  InitialCondition=vinit  SampleTime=-1  HasFrameUpgradeWarning=on
  FixPt Relational Operator : RelationalOperator  Operator=>  OutDataTypeStr=boolean  ZeroCross=off  InputSameDT=off
  Positive : Subsystem  mask(Compare To Zero){relop=>, OutDataTypeStr=boolean, ZeroCross=off}
      mask prompts: relop "Simulink:masks:Operator_MP"; OutDataTypeStr "Simulink:masks:OutputDataType_MP"; ZeroCross "Simulink:masks:EnableZerocrossingDetection_MP"
      mask help: Simulink:masks:CompareToZero_MD
      mask init:
      | OutDataTypeStr = 'boolean';
      | ZeroCross = 'off';
      | blkName = 'parallel_8_min_cost_function/Min_cost_function_and_vopt1/Detect Rise\nPositive/Positive';
      | relop = '>';
      | setValue = 'boolean';
      mask TypeOptions relop: == | ~= | < | <= | >= | >
      mask TypeOptions OutDataTypeStr: Simulink:masks:uint8 | Simulink:masks:boolean
      mask Callback ZeroCross: sl('zeroCrossEnable', gcbh);
      mask Display: disp([relop,' 0'])
  Y : Outport  SampleTime=1e-08
  wires:
  U/1 -> Positive/1(u)
  Delay Input1/1 -> FixPt Relational Operator/2
  FixPt Relational Operator/1 -> Y/1
  Positive/1(y) -> FixPt Relational Operator/1, Delay Input1/1

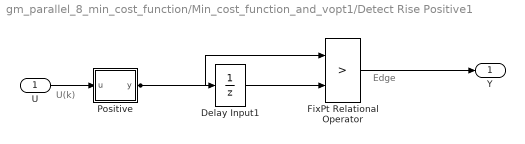
== system gm_parallel_8_min_cost_function/Min_cost_function_and_vopt1/Detect Rise Positive1 ==
  note: Edge
  note: U(k)
  U : Inport  OutDataTypeStr=boolean  SampleTime=1e-08
  Delay Input1 : UnitDelay  Description=Store in Global RAM  DisableCoverage=on  InitialCondition=vinit  SampleTime=-1  HasFrameUpgradeWarning=on
  FixPt Relational Operator : RelationalOperator  Operator=>  OutDataTypeStr=boolean  ZeroCross=off  InputSameDT=off
  Positive : Subsystem  mask(Compare To Zero){relop=>, OutDataTypeStr=boolean, ZeroCross=off}
      mask prompts: relop "Simulink:masks:Operator_MP"; OutDataTypeStr "Simulink:masks:OutputDataType_MP"; ZeroCross "Simulink:masks:EnableZerocrossingDetection_MP"
      mask help: Simulink:masks:CompareToZero_MD
      mask init:
      | OutDataTypeStr = 'boolean';
      | ZeroCross = 'off';
      | blkName = 'parallel_8_min_cost_function/Min_cost_function_and_vopt1/Detect Rise\nPositive1/Positive';
      | relop = '>';
      | setValue = 'boolean';
      mask TypeOptions relop: == | ~= | < | <= | >= | >
      mask TypeOptions OutDataTypeStr: Simulink:masks:uint8 | Simulink:masks:boolean
      mask Callback ZeroCross: sl('zeroCrossEnable', gcbh);
      mask Display: disp([relop,' 0'])
  Y : Outport  SampleTime=1e-08
  wires:
  U/1 -> Positive/1(u)
  Delay Input1/1 -> FixPt Relational Operator/2
  FixPt Relational Operator/1 -> Y/1
  Positive/1(y) -> FixPt Relational Operator/1, Delay Input1/1
